simulink model "abs_relay"  (R2012b)
settings: Solver=ode5  SolverMode=SingleTasking  StartTime=0.0  StopTime=15  FixedStep=0.01  RelTol=1e-3  AbsTol=1e-6
undefined symbols (not defined in the file): abspositionscale, abspowerscale, abstemperaturescale, absvelocityscale, RTDAC4PCIBaseAddress
libraries: simulink_extras x2
settings Model: SimulationMode=external  ExtModeTrigDuration=6000  Creator=jims  LastModifiedBy=inteco
settings DataIOCC: ExternalInput=[]  InitialState=[]  LimitDataPoints=off  MaxDataPoints=5000  SignalLoggingSaveFormat=ModelDataLogs  SaveOutput=off  SaveTime=off  SignalLoggingName=sigsOut
settings OptimizationCC: BlockReduction=off  BooleanDataType=off  InitFltsAndDblsToZero=on
settings DebuggingCC: SaveWithParameterizedLinksMsg=none  SignalResolutionControl=TryResolveAllWithWarning  SolverPrmCheckMsg=none  MultiTaskDSMMsg=warning  MultiTaskCondExecSysMsg=none  IntegerOverflowMsg=none  FcnCallInpInsideContextMsg=UseLocalSettings  StrictBusMsg=None
settings HardwareCC: ProdIntDivRoundTo=Zero  ProdEndianess=LittleEndian  ProdHWDeviceType=Generic->32-bit x86 compatible  TargetEndianess=LittleEndian  TargetHWDeviceType=MATLAB Host
settings RTWCC: SystemTargetFile=rtwin.tlc  TemplateMakefile=rtwin.tmf  Description=Real-Time Windows Target  ProcessScript=rtwin_make_rtw_hook  IncludeERTFirstTime=on  RTWCompilerOptimization=On
settings CodeAppCC: MaxIdLength=95
settings RTWinTargetCC: TargetLibSuffix=_rtwin.lib  TargetPreCompLibLocation=E:\apps_W64\MATLAB\x64_R2012b\toolbox\rtw\targets\rtwin\lib\win64  CodeReplacementLibrary=ANSI_C  RTWinDir=E:/apps_W64/MATLAB/X64_R2~1/toolbox/rtw/targets/rtwin  TargetArch=win64

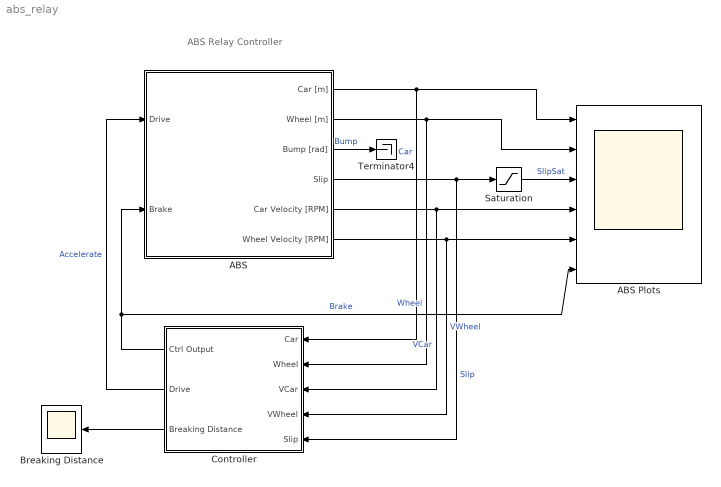
== system abs_relay ==
  note: ABS Relay Controller
  ABS : Subsystem  mask{BaseAddress=RTDAC4PCIBaseAddress(-1,-1), T0=0.01}
      mask prompts: BaseAddress "Base Address"; T0 "Sample Time"
      mask Display: image(imread('abs.bmp'))
  ABS Plots : Scope  NumInputPorts=6
      settings: TimeRange=15  YMin=0~0~-2~0~0~0  YMax=200~200~2~3000~3000~1  SaveName=ABSHistory1  MaxDataPoints=6000
  Breaking Distance : Scope
      settings: TimeRange=20  YMin=0  YMax=15  SaveName=ABSBreakingWay  MaxDataPoints=6000
  Controller : Subsystem  mask(ABS Relay Controller){VelTr=1700, SwPoint=[0.3 0.3], CntLevel=[0 0.4]}
      mask prompts: VelTr "Velocity Treshold [RPM]:"; SwPoint "Switch Point [ON OFF]:"; CntLevel "Control When [ON OFF]:"
      mask help: Parameters of the ABS relay controller
  Saturation : Saturate  UpperLimit=1.5  LowerLimit=-1.5
  Terminator4 : Terminator
  wires:
  Controller/2(Drive) -> ABS/1(Drive)  "Accelerate"
  Controller/1(Ctrl Output) -> ABS Plots/6, ABS/2(Brake)  "Brake"
  ABS/1(Car [m]) -> Controller/1(Car), ABS Plots/1  "Car"
  ABS/2(Wheel [m]) -> Controller/2(Wheel), ABS Plots/2  "Wheel"
  ABS/5(Car Velocity [RPM]) -> Controller/3(VCar), ABS Plots/4  "VCar"
  ABS/6(Wheel Velocity [RPM]) -> Controller/4(VWheel), ABS Plots/5  "VWheel"
  ABS/4(Slip) -> Controller/5(Slip), Saturation/1  "Slip"
  Controller/3(Breaking Distance) -> Breaking Distance/1
  Saturation/1 -> ABS Plots/3  "SlipSat"
  ABS/3(Bump [rad]) -> Terminator4/1  "Bump"

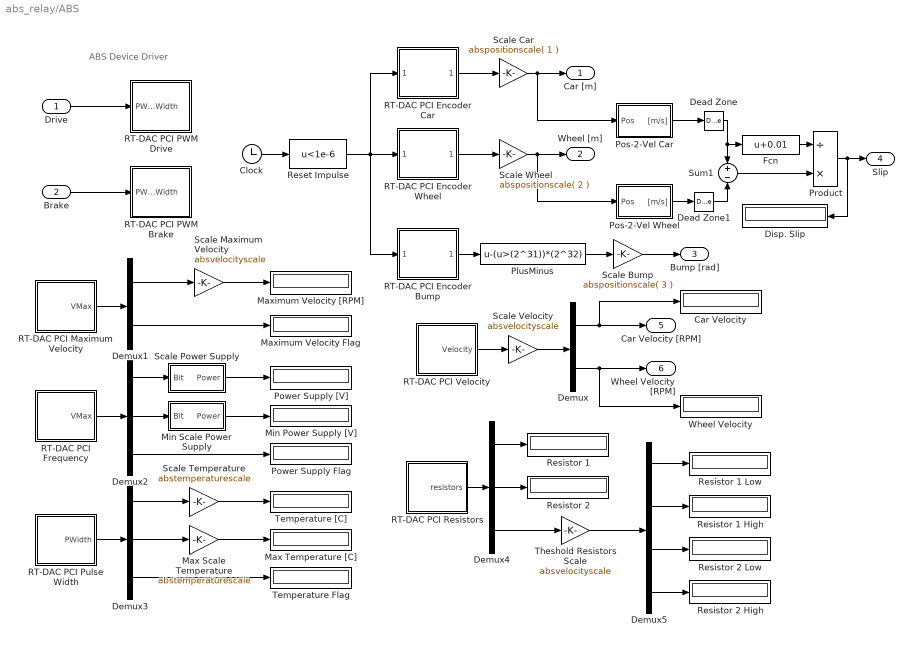
== system abs_relay/ABS ==
  note: ABS Device Driver
  Drive : Inport
  Brake : Inport  Port=2
  Car Velocity : Display
  Clock : Clock
  Dead Zone : DeadZone  LowerValue=-0.05  UpperValue=0.05  SaturateOnIntegerOverflow=on
  Dead Zone1 : DeadZone  LowerValue=-0.05  UpperValue=0.05  SaturateOnIntegerOverflow=on
  Demux : Demux  Outputs=2
  Demux1 : Demux  Outputs=2
  Demux2 : Demux  Outputs=3
  Demux3 : Demux  Outputs=3
  Demux4 : Demux  Outputs=[1 1 4]
  Demux5 : Demux
  Disp. Slip : Display
      settings: Format=bank
  Fcn : Fcn  Expr=u+0.01
  Max Scale Temperature : Gain  Gain=abstemperaturescale  OutDataTypeStr=Inherit: Same as input  ParamDataTypeStr=Inherit: Same as input
  Max Temperature [C] : Display
  Maximum Velocity Flag : Display
  Maximum Velocity [RPM] : Display
  Min Power Supply [V] : Display
  Min Scale Power Supply : Subsystem
  PlusMinus : Fcn  Expr=u-(u>(2^31))*(2^32)
  Pos-2-Vel Car : Subsystem
  Pos-2-Vel Wheel : Subsystem
  Power Supply Flag : Display
  Power Supply [V] : Display
  Product : Product  Inputs=/*  SaturateOnIntegerOverflow=on  InputSameDT=on  OutDataTypeStr=Inherit: Same as first input
  RT-DAC PCI Encoder Bump : Subsystem  mask(Incremental Encoders){BaseAddress=BaseAddress, ChannelIdx=2, T0=T0}
      mask prompts: BaseAddress "Base Address:"; ChannelIdx "Channel:"; T0 "Sample Time (sec):"
      mask help: RT-DAC PCI Device Driver
      mask Help: Set up each field for your specific hardware configuration.
      mask TypeOptions ChannelIdx: 0 | 1 | 2 | 3
      mask Display: plot(0,0,100,100,[90,80,80,11,11],[90,90,20,20,80],[11,80],[80,80],[80,80],[20,14],[80,85,85,80],[45,45,66,66],[45,45,74,74],[20,13,13,20],[15,27,27,15,15],[75,75,26,26,75],[33,48,48,33,33],[75,75,55,55,75],[55,55,71,71,55],[55,75,75,55,55],[33,41,41,33,33],[50,50,27,27,50],[48,56,56,48,48],[50,50,27,27,50],[62,70,70,62,62],[50,50,27,27,50])
  RT-DAC PCI Encoder Car : Subsystem  mask(Incremental Encoders){BaseAddress=BaseAddress, ChannelIdx=0, T0=T0}
      mask prompts: BaseAddress "Base Address:"; ChannelIdx "Channel:"; T0 "Sample Time (sec):"
      mask help: RT-DAC PCI Device Driver
      mask Help: Set up each field for your specific hardware configuration.
      mask TypeOptions ChannelIdx: 0 | 1 | 2 | 3
      mask Display: plot(0,0,100,100,[90,80,80,11,11],[90,90,20,20,80],[11,80],[80,80],[80,80],[20,14],[80,85,85,80],[45,45,66,66],[45,45,74,74],[20,13,13,20],[15,27,27,15,15],[75,75,26,26,75],[33,48,48,33,33],[75,75,55,55,75],[55,55,71,71,55],[55,75,75,55,55],[33,41,41,33,33],[50,50,27,27,50],[48,56,56,48,48],[50,50,27,27,50],[62,70,70,62,62],[50,50,27,27,50])
  RT-DAC PCI Encoder Wheel : Subsystem  mask(Incremental Encoders){BaseAddress=BaseAddress, ChannelIdx=1, T0=T0}
      mask prompts: BaseAddress "Base Address:"; ChannelIdx "Channel:"; T0 "Sample Time (sec):"
      mask help: RT-DAC PCI Device Driver
      mask Help: Set up each field for your specific hardware configuration.
      mask TypeOptions ChannelIdx: 0 | 1 | 2 | 3
      mask Display: plot(0,0,100,100,[90,80,80,11,11],[90,90,20,20,80],[11,80],[80,80],[80,80],[20,14],[80,85,85,80],[45,45,66,66],[45,45,74,74],[20,13,13,20],[15,27,27,15,15],[75,75,26,26,75],[33,48,48,33,33],[75,75,55,55,75],[55,55,71,71,55],[55,75,75,55,55],[33,41,41,33,33],[50,50,27,27,50],[48,56,56,48,48],[50,50,27,27,50],[62,70,70,62,62],[50,50,27,27,50])
  RT-DAC PCI Frequency : Subsystem  mask(Incremental Encoders){BaseAddress=BaseAddress, T0=T0}
      mask prompts: BaseAddress "Base Address:"; T0 "Sample Time (sec):"
      mask help: RT-DAC PCI Device Driver
      mask Help: Set up each field for your specific hardware configuration.
      mask Display: plot(0,0,100,100,[90,80,80,11,11],[90,90,20,20,80],[11,80],[80,80],[80,80],[20,14],[80,85,85,80],[45,45,66,66],[45,45,74,74],[20,13,13,20],[15,27,27,15,15],[75,75,26,26,75],[33,48,48,33,33],[75,75,55,55,75],[55,55,71,71,55],[55,75,75,55,55],[33,41,41,33,33],[50,50,27,27,50],[48,56,56,48,48],[50,50,27,27,50],[62,70,70,62,62],[50,50,27,27,50])
  RT-DAC PCI Maximum Velocity : Subsystem  mask(Incremental Encoders){BaseAddress=BaseAddress, T0=T0}
      mask prompts: BaseAddress "Base Address:"; T0 "Sample Time (sec):"
      mask help: RT-DAC PCI Device Driver
      mask Help: Set up each field for your specific hardware configuration.
      mask Display: plot(0,0,100,100,[90,80,80,11,11],[90,90,20,20,80],[11,80],[80,80],[80,80],[20,14],[80,85,85,80],[45,45,66,66],[45,45,74,74],[20,13,13,20],[15,27,27,15,15],[75,75,26,26,75],[33,48,48,33,33],[75,75,55,55,75],[55,55,71,71,55],[55,75,75,55,55],[33,41,41,33,33],[50,50,27,27,50],[48,56,56,48,48],[50,50,27,27,50],[62,70,70,62,62],[50,50,27,27,50])
  RT-DAC PCI PWM Brake : Subsystem  mask(PWM Module){BaseAddress=BaseAddress, ChanIdx=1, ChanMode=8 Bit, ChanPresc=7, SetOutputsFlag=on, SetOutputsValue=0, T0=T0}
      mask prompts: BaseAddress "IO Base Address:"; ChanIdx "Channel:"; ChanMode "Channel Mode:"; ChanPresc "Channel Prescaler:"; SetOutputsFlag "Set Outputs At Termination"; SetOutputsValue "Termination Outputs:"; T0 "Sample Time (sec):"
      mask help: RT-DAC PCI Device Driver
      mask Help: Set up each field for your specific hardware configuration.
      mask TypeOptions ChanIdx: 0 | 1 | 2 | 3
      mask TypeOptions ChanMode: 8 Bit | 12 Bit
      mask Display: plot(0,0,100,100,[90,80,80,11,11],[90,90,20,20,80],[11,80],[80,80],[80,80],[20,14],[80,85,85,80],[45,45,66,66],[45,45,74,74],[20,13,13,20],[15,27,27,15,15],[75,75,26,26,75],[33,48,48,33,33],[75,75,55,55,75],[55,55,71,71,55],[55,75,75,55,55],[33,41,41,33,33],[50,50,27,27,50],[48,56,56,48,48],[50,50,27,27,50],[62,70,70,62,62],[50,50,27,27,50])
  RT-DAC PCI PWM Drive : Subsystem  mask(PWM Module){BaseAddress=BaseAddress, ChanIdx=0, ChanMode=8 Bit, ChanPresc=7, SetOutputsFlag=on, SetOutputsValue=0, T0=T0}
      mask prompts: BaseAddress "IO Base Address:"; ChanIdx "Channel:"; ChanMode "Channel Mode:"; ChanPresc "Channel Prescaler:"; SetOutputsFlag "Set Outputs At Termination"; SetOutputsValue "Termination Outputs:"; T0 "Sample Time (sec):"
      mask help: RT-DAC PCI Device Driver
      mask Help: Set up each field for your specific hardware configuration.
      mask TypeOptions ChanIdx: 0 | 1 | 2 | 3
      mask TypeOptions ChanMode: 8 Bit | 12 Bit
      mask Display: plot(0,0,100,100,[90,80,80,11,11],[90,90,20,20,80],[11,80],[80,80],[80,80],[20,14],[80,85,85,80],[45,45,66,66],[45,45,74,74],[20,13,13,20],[15,27,27,15,15],[75,75,26,26,75],[33,48,48,33,33],[75,75,55,55,75],[55,55,71,71,55],[55,75,75,55,55],[33,41,41,33,33],[50,50,27,27,50],[48,56,56,48,48],[50,50,27,27,50],[62,70,70,62,62],[50,50,27,27,50])
  RT-DAC PCI Pulse Width : Subsystem  mask(Incremental Encoders){BaseAddress=BaseAddress, T0=T0}
      mask prompts: BaseAddress "Base Address:"; T0 "Sample Time (sec):"
      mask help: RT-DAC PCI Device Driver
      mask Help: Set up each field for your specific hardware configuration.
      mask Display: plot(0,0,100,100,[90,80,80,11,11],[90,90,20,20,80],[11,80],[80,80],[80,80],[20,14],[80,85,85,80],[45,45,66,66],[45,45,74,74],[20,13,13,20],[15,27,27,15,15],[75,75,26,26,75],[33,48,48,33,33],[75,75,55,55,75],[55,55,71,71,55],[55,75,75,55,55],[33,41,41,33,33],[50,50,27,27,50],[48,56,56,48,48],[50,50,27,27,50],[62,70,70,62,62],[50,50,27,27,50])
  RT-DAC PCI Resistors : Subsystem  mask(Incremental Encoders){BaseAddress=BaseAddress, T0=T0}
      mask prompts: BaseAddress "Base Address:"; T0 "Sample Time (sec):"
      mask help: RT-DAC PCI Device Driver
      mask Help: Set up each field for your specific hardware configuration.
      mask Display: plot(0,0,100,100,[90,80,80,11,11],[90,90,20,20,80],[11,80],[80,80],[80,80],[20,14],[80,85,85,80],[45,45,66,66],[45,45,74,74],[20,13,13,20],[15,27,27,15,15],[75,75,26,26,75],[33,48,48,33,33],[75,75,55,55,75],[55,55,71,71,55],[55,75,75,55,55],[33,41,41,33,33],[50,50,27,27,50],[48,56,56,48,48],[50,50,27,27,50],[62,70,70,62,62],[50,50,27,27,50])
  RT-DAC PCI Velocity : Subsystem  mask(Incremental Encoders){BaseAddress=BaseAddress, T0=T0}
      mask prompts: BaseAddress "Base Address:"; T0 "Sample Time (sec):"
      mask help: RT-DAC PCI Device Driver
      mask Help: Set up each field for your specific hardware configuration.
      mask Display: plot(0,0,100,100,[90,80,80,11,11],[90,90,20,20,80],[11,80],[80,80],[80,80],[20,14],[80,85,85,80],[45,45,66,66],[45,45,74,74],[20,13,13,20],[15,27,27,15,15],[75,75,26,26,75],[33,48,48,33,33],[75,75,55,55,75],[55,55,71,71,55],[55,75,75,55,55],[33,41,41,33,33],[50,50,27,27,50],[48,56,56,48,48],[50,50,27,27,50],[62,70,70,62,62],[50,50,27,27,50])
  Reset Impulse : Fcn  Expr=u<1e-6
  Resistor 1 : Display
  Resistor 1 High : Display
  Resistor 1 Low : Display
  Resistor 2 : Display
  Resistor 2 High : Display
  Resistor 2 Low : Display
  Scale Bump : Gain  Gain=abspositionscale( 3 )  OutDataTypeStr=Inherit: Same as input  ParamDataTypeStr=Inherit: Same as input
  Scale Car : Gain  Gain=abspositionscale( 1 )  OutDataTypeStr=Inherit: Same as input  ParamDataTypeStr=Inherit: Same as input
  Scale Maximum Velocity : Gain  Gain=absvelocityscale  OutDataTypeStr=Inherit: Same as input  ParamDataTypeStr=Inherit: Same as input
  Scale Velocity : Gain  Gain=absvelocityscale  OutDataTypeStr=Inherit: Same as input  ParamDataTypeStr=Inherit: Same as input
  Scale Wheel : Gain  Gain=abspositionscale( 2 )  OutDataTypeStr=Inherit: Same as input  ParamDataTypeStr=Inherit: Same as input
  Scale Power Supply : Subsystem
  Scale Temperature : Gain  Gain=abstemperaturescale  OutDataTypeStr=Inherit: Same as input  ParamDataTypeStr=Inherit: Same as input
  Sum1 : Sum  Inputs=+-  SaturateOnIntegerOverflow=on  InputSameDT=on  OutDataTypeStr=Inherit: Same as first input
  Temperature Flag : Display
  Temperature [C] : Display
  Theshold Resistors Scale : Gain  Gain=absvelocityscale  OutDataTypeStr=Inherit: Same as input  ParamDataTypeStr=Inherit: Same as input
  Wheel Velocity : Display
  Car [m] : Outport
  Wheel [m] : Outport  Port=2
  Bump [rad] : Outport  Port=3
  Slip : Outport  Port=4
  Car Velocity [RPM] : Outport  Port=5
  Wheel Velocity [RPM] : Outport  Port=6
  wires:
  PlusMinus/1 -> Scale Bump/1
  RT-DAC PCI Encoder Car/1(Encoder Counter) -> Scale Car/1
  RT-DAC PCI Encoder Wheel/1(Encoder Counter) -> Scale Wheel/1
  RT-DAC PCI Encoder Bump/1(Encoder Counter) -> PlusMinus/1
  Scale Car/1 -> Car [m]/1, Pos-2-Vel Car/1(Pos)
  Scale Wheel/1 -> Wheel [m]/1, Pos-2-Vel Wheel/1(Pos)
  Scale Bump/1 -> Bump [rad]/1
  RT-DAC PCI Velocity/1(Velocity) -> Scale Velocity/1
  Scale Velocity/1 -> Demux/1
  Scale Power Supply/1(Power) -> Power Supply [V]/1
  Scale Temperature/1 -> Temperature [C]/1
  Drive/1 -> RT-DAC PCI PWM Drive/1(PWM Width)
  Brake/1 -> RT-DAC PCI PWM Brake/1(PWM Width)
  Demux/1 -> Car Velocity [RPM]/1, Car Velocity/1
  Demux/2 -> Wheel Velocity [RPM]/1, Wheel Velocity/1
  RT-DAC PCI Maximum Velocity/1(VMax) -> Demux1/1
  Demux1/1 -> Scale Maximum Velocity/1
  Scale Maximum Velocity/1 -> Maximum Velocity [RPM]/1
  Demux1/2 -> Maximum Velocity Flag/1
  RT-DAC PCI Frequency/1(VMax) -> Demux2/1
  Demux2/1 -> Scale Power Supply/1(Bit)
  RT-DAC PCI Pulse Width/1(PWidth) -> Demux3/1
  Demux3/1 -> Scale Temperature/1
  Clock/1 -> Reset Impulse/1
  Reset Impulse/1 -> RT-DAC PCI Encoder Wheel/1(Reset), RT-DAC PCI Encoder Car/1(Reset), RT-DAC PCI Encoder Bump/1(Reset)
  Demux2/2 -> Min Scale Power Supply/1(Bit)
  Min Scale Power Supply/1(Power) -> Min Power Supply [V]/1
  Demux2/3 -> Power Supply Flag/1
  Max Scale Temperature/1 -> Max Temperature [C]/1
  Demux3/2 -> Max Scale Temperature/1
  Demux3/3 -> Temperature Flag/1
  RT-DAC PCI Resistors/1(resistors) -> Demux4/1
  Demux4/1 -> Resistor 1/1
  Demux4/2 -> Resistor 2/1
  Demux4/3 -> Theshold Resistors Scale/1
  Theshold Resistors Scale/1 -> Demux5/1
  Demux5/1 -> Resistor 1 Low/1
  Demux5/2 -> Resistor 1 High/1
  Demux5/3 -> Resistor 2 Low/1
  Demux5/4 -> Resistor 2 High/1
  Sum1/1 -> Product/2
  Fcn/1 -> Product/1
  Product/1 -> Slip/1, Disp. Slip/1
  Pos-2-Vel Wheel/1("[m/s]") -> Dead Zone1/1
  Pos-2-Vel Car/1("[m/s]") -> Dead Zone/1
  Dead Zone/1 -> Sum1/1, Fcn/1
  Dead Zone1/1 -> Sum1/2

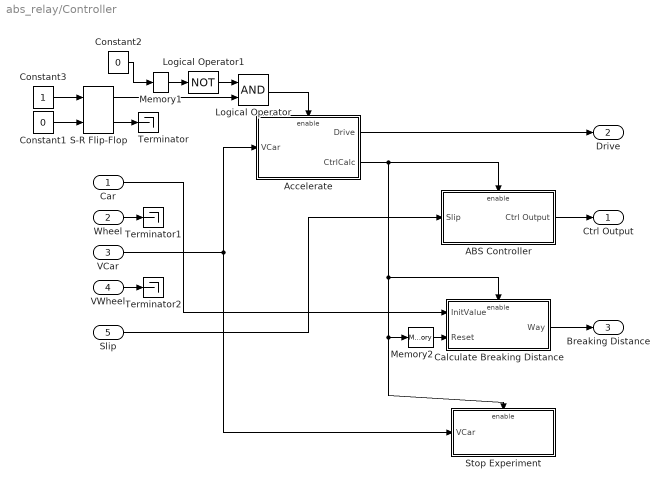
== system abs_relay/Controller ==
  Car : Inport
  Wheel : Inport  Port=2
  VCar : Inport  Port=3
  VWheel : Inport  Port=4
  Slip : Inport  Port=5
  ABS Controller : Subsystem  TreatAsAtomicUnit=on
  Accelerate : Subsystem  TreatAsAtomicUnit=on
  Calculate Breaking Distance : Subsystem  TreatAsAtomicUnit=on
  Constant1 : Constant  Value=0
  Constant2 : Constant  Value=0
  Constant3 : Constant
  Logical Operator : Logic
  Logical Operator1 : Logic  Operator=NOT
  Memory1 : Memory
  Memory2 : Memory
  S-R Flip-Flop : simulink_extras/Flip Flops/S-R Flip-Flop  initial_condition=0
  Stop Experiment : Subsystem  TreatAsAtomicUnit=on
  Terminator : Terminator
  Terminator1 : Terminator
  Terminator2 : Terminator
  Ctrl Output : Outport
  Drive : Outport  Port=2
  Breaking Distance : Outport  Port=3
  wires:
  Logical Operator1/1 -> Logical Operator/1
  S-R Flip-Flop/1 -> Logical Operator/2
  Logical Operator/1 -> Accelerate/Enable
  Accelerate/2(CtrlCalc) -> ABS Controller/Enable, Calculate Breaking Distance/Enable, Memory2/1, Stop Experiment/Enable
  S-R Flip-Flop/2 -> Terminator/1
  Constant1/1 -> S-R Flip-Flop/2
  Accelerate/1(Drive) -> Drive/1
  ABS Controller/1(Ctrl Output) -> Ctrl Output/1
  Calculate Breaking Distance/1(Way) -> Breaking Distance/1
  VCar/1 -> Accelerate/1(VCar), Stop Experiment/1(VCar)
  Car/1 -> Calculate Breaking Distance/1(InitValue)
  Memory2/1 -> Calculate Breaking Distance/2(Reset)
  Memory1/1 -> Logical Operator1/1
  Slip/1 -> ABS Controller/1(Slip)
  Constant2/1 -> Memory1/1
  Constant3/1 -> S-R Flip-Flop/1
  Wheel/1 -> Terminator1/1
  VWheel/1 -> Terminator2/1

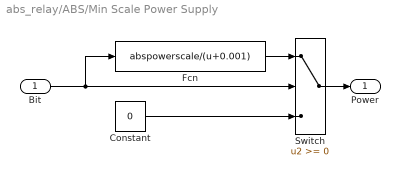
== system abs_relay/ABS/Min Scale Power Supply ==
  Bit : Inport
  Constant : Constant  Value=0
  Fcn : Fcn  Expr=abspowerscale/(u+0.001)
  Switch : Switch  SaturateOnIntegerOverflow=on  InputSameDT=on
  Power : Outport
  wires:
  Constant/1 -> Switch/3
  Fcn/1 -> Switch/1
  Switch/1 -> Power/1
  Bit/1 -> Fcn/1, Switch/2

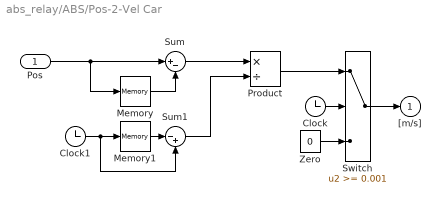
== system abs_relay/ABS/Pos-2-Vel Car ==
  Pos : Inport
  Clock : Clock
  Clock1 : Clock
  Memory : Memory  InheritSampleTime=on
  Memory1 : Memory  InheritSampleTime=on
  Product : Product  Inputs=*/  SaturateOnIntegerOverflow=on  InputSameDT=on  OutDataTypeStr=Inherit: Same as first input
  Sum : Sum  Inputs=|+-  SaturateOnIntegerOverflow=on  InputSameDT=on  OutDataTypeStr=Inherit: Same as first input
  Sum1 : Sum  Inputs=|-+  SaturateOnIntegerOverflow=on  InputSameDT=on  OutDataTypeStr=Inherit: Same as first input
  Switch : Switch  Threshold=0.001  SaturateOnIntegerOverflow=on  InputSameDT=on
  Zero : Constant  Value=0
  "[m/s]" : Outport
  wires:
  Sum1/1 -> Product/2
  Memory1/1 -> Sum1/1
  Clock1/1 -> Sum1/2, Memory1/1
  Sum/1 -> Product/1
  Product/1 -> Switch/1
  Zero/1 -> Switch/3
  Switch/1 -> "[m/s]"/1
  Clock/1 -> Switch/2
  Memory/1 -> Sum/2
  Pos/1 -> Sum/1, Memory/1

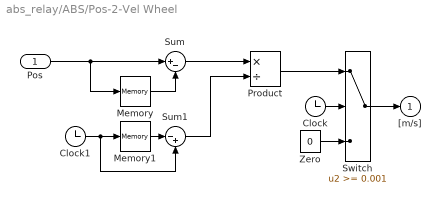
== system abs_relay/ABS/Pos-2-Vel Wheel ==
  Pos : Inport
  Clock : Clock
  Clock1 : Clock
  Memory : Memory  InheritSampleTime=on
  Memory1 : Memory  InheritSampleTime=on
  Product : Product  Inputs=*/  SaturateOnIntegerOverflow=on  InputSameDT=on  OutDataTypeStr=Inherit: Same as first input
  Sum : Sum  Inputs=|+-  SaturateOnIntegerOverflow=on  InputSameDT=on  OutDataTypeStr=Inherit: Same as first input
  Sum1 : Sum  Inputs=|-+  SaturateOnIntegerOverflow=on  InputSameDT=on  OutDataTypeStr=Inherit: Same as first input
  Switch : Switch  Threshold=0.001  SaturateOnIntegerOverflow=on  InputSameDT=on
  Zero : Constant  Value=0
  "[m/s]" : Outport
  wires:
  Pos/1 -> Memory/1, Sum/1
  Memory/1 -> Sum/2
  Clock/1 -> Switch/2
  Switch/1 -> "[m/s]"/1
  Zero/1 -> Switch/3
  Product/1 -> Switch/1
  Sum/1 -> Product/1
  Clock1/1 -> Memory1/1, Sum1/2
  Memory1/1 -> Sum1/1
  Sum1/1 -> Product/2

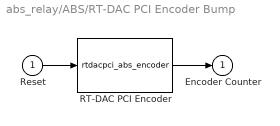
== system abs_relay/ABS/RT-DAC PCI Encoder Bump ==
  Reset : Inport
  RT-DAC PCI Encoder : S-Function  FunctionName=rtdacpci_abs_encoder  Parameters=BaseAddress, ChannelIdx, T0  EnableBusSupport=off
  Encoder Counter : Outport
  wires:
  Reset/1 -> RT-DAC PCI Encoder/1
  RT-DAC PCI Encoder/1 -> Encoder Counter/1

== system abs_relay/ABS/RT-DAC PCI Encoder Car ==
  Reset : Inport
  RT-DAC PCI Encoder : S-Function  FunctionName=rtdacpci_abs_encoder  Parameters=BaseAddress, ChannelIdx, T0  EnableBusSupport=off
  Encoder Counter : Outport
  wires:
  Reset/1 -> RT-DAC PCI Encoder/1
  RT-DAC PCI Encoder/1 -> Encoder Counter/1

== system abs_relay/ABS/RT-DAC PCI Encoder Wheel ==
  Reset : Inport
  RT-DAC PCI Encoder : S-Function  FunctionName=rtdacpci_abs_encoder  Parameters=BaseAddress, ChannelIdx, T0  EnableBusSupport=off
  Encoder Counter : Outport
  wires:
  RT-DAC PCI Encoder/1 -> Encoder Counter/1
  Reset/1 -> RT-DAC PCI Encoder/1

== system abs_relay/ABS/RT-DAC PCI Frequency ==
  RT-DAC PCI Frequency : S-Function  FunctionName=rtdacpci_abs_frequency  Parameters=BaseAddress, T0  EnableBusSupport=off
  VMax : Outport
  wires:
  RT-DAC PCI Frequency/1 -> VMax/1

== system abs_relay/ABS/RT-DAC PCI Maximum Velocity ==
  RT-DAC PCI VMax : S-Function  FunctionName=rtdacpci_abs_vmax  Parameters=BaseAddress, T0  EnableBusSupport=off
  VMax : Outport
  wires:
  RT-DAC PCI VMax/1 -> VMax/1

== system abs_relay/ABS/RT-DAC PCI PWM Brake ==
  PWM Width : Inport
  "RT-DAC PCI PWM " : S-Function  FunctionName=rtdacpci_abs_pwm  Parameters=BaseAddress, ChanIdx, ChanMode, ChanPresc, SetOutputsFlag, SetOutputsValue, T0  EnableBusSupport=off
  wires:
  PWM Width/1 -> "RT-DAC PCI PWM "/1

== system abs_relay/ABS/RT-DAC PCI PWM Drive ==
  PWM Width : Inport
  "RT-DAC PCI PWM " : S-Function  FunctionName=rtdacpci_abs_pwm  Parameters=BaseAddress, ChanIdx, ChanMode, ChanPresc, SetOutputsFlag, SetOutputsValue, T0  EnableBusSupport=off
  wires:
  PWM Width/1 -> "RT-DAC PCI PWM "/1

== system abs_relay/ABS/RT-DAC PCI Pulse Width ==
  RT-DAC PCI Pulse Width : S-Function  FunctionName=rtdacpci_abs_pulsewidth  Parameters=BaseAddress, T0  EnableBusSupport=off
  PWidth : Outport
  wires:
  RT-DAC PCI Pulse Width/1 -> PWidth/1

== system abs_relay/ABS/RT-DAC PCI Resistors ==
  RT-DAC PCI Resistors : S-Function  FunctionName=rtdacpci_abs_resistors  Parameters=BaseAddress, T0  EnableBusSupport=off
  resistors : Outport
  wires:
  RT-DAC PCI Resistors/1 -> resistors/1

== system abs_relay/ABS/RT-DAC PCI Velocity ==
  RT-DAC PCI Velocity : S-Function  FunctionName=rtdacpci_abs_velocity  Parameters=BaseAddress, T0  EnableBusSupport=off
  Velocity : Outport
  wires:
  RT-DAC PCI Velocity/1 -> Velocity/1

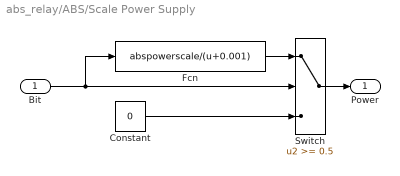
== system abs_relay/ABS/Scale Power Supply ==
  Bit : Inport
  Constant : Constant  Value=0
  Fcn : Fcn  Expr=abspowerscale/(u+0.001)
  Switch : Switch  Threshold=0.5  SaturateOnIntegerOverflow=on  InputSameDT=on
  Power : Outport
  wires:
  Bit/1 -> Switch/2, Fcn/1
  Switch/1 -> Power/1
  Fcn/1 -> Switch/1
  Constant/1 -> Switch/3

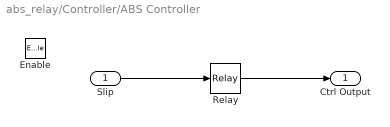
== system abs_relay/Controller/ABS Controller ==
  Slip : Inport
  Enable : EnablePort  PropagateVarSize=During execution
  Relay : Relay  OnSwitchValue=SwPoint(1)  OffSwitchValue=SwPoint(2)  OnOutputValue=CntLevel(1)  OffOutputValue=CntLevel(2)
  Ctrl Output : Outport
  wires:
  Slip/1 -> Relay/1
  Relay/1 -> Ctrl Output/1

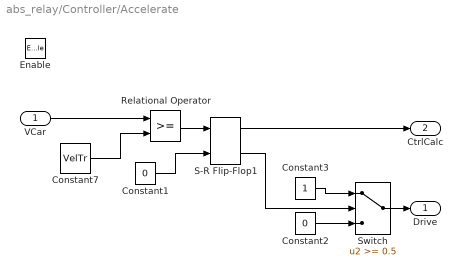
== system abs_relay/Controller/Accelerate ==
  VCar : Inport
  Enable : EnablePort  PropagateVarSize=During execution
  Constant1 : Constant  Value=0
  Constant2 : Constant  Value=0
  Constant3 : Constant
  Constant7 : Constant  Value=VelTr
  Relational Operator : RelationalOperator  InputSameDT=on
  S-R Flip-Flop1 : simulink_extras/Flip Flops/S-R Flip-Flop  initial_condition=0
  Switch : Switch  Threshold=0.5  SaturateOnIntegerOverflow=on  InputSameDT=on
  Drive : Outport
  CtrlCalc : Outport  Port=2
  wires:
  Constant7/1 -> Relational Operator/2
  Relational Operator/1 -> S-R Flip-Flop1/1
  VCar/1 -> Relational Operator/1
  Constant1/1 -> S-R Flip-Flop1/2
  Switch/1 -> Drive/1
  S-R Flip-Flop1/2 -> Switch/2
  Constant2/1 -> Switch/3
  S-R Flip-Flop1/1 -> CtrlCalc/1
  Constant3/1 -> Switch/1

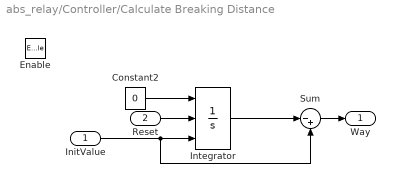
== system abs_relay/Controller/Calculate Breaking Distance ==
  InitValue : Inport
  Reset : Inport  Port=2
  Enable : EnablePort  PropagateVarSize=During execution
  Constant2 : Constant  Value=0
  Integrator : Integrator  ExternalReset=rising  InitialConditionSource=external
  Sum : Sum  Inputs=|-+  SaturateOnIntegerOverflow=on  InputSameDT=on  OutDataTypeStr=Inherit: Same as first input
  Way : Outport
  wires:
  Constant2/1 -> Integrator/1
  Integrator/1 -> Sum/1
  InitValue/1 -> Sum/2, Integrator/3
  Reset/1 -> Integrator/2
  Sum/1 -> Way/1

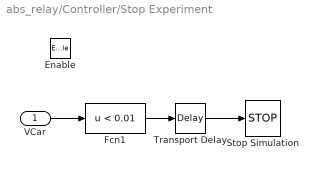
== system abs_relay/Controller/Stop Experiment ==
  VCar : Inport
  Enable : EnablePort  PropagateVarSize=During execution
  Fcn1 : Fcn  Expr=u < 0.01
  Stop Simulation : Stop
  Transport Delay : TransportDelay  DelayTime=0.5  FixedBuffer=on
  wires:
  Fcn1/1 -> Transport Delay/1
  Transport Delay/1 -> Stop Simulation/1
  VCar/1 -> Fcn1/1
